simulink model "statdynamic"  (R2019b)
settings: Solver=ode45  StartTime=0.0  StopTime=100  MaxStep=0.0001  RelTol=1e-3
libraries: simulink x5
settings Model: Creator=Roman  LastModifiedBy=romak

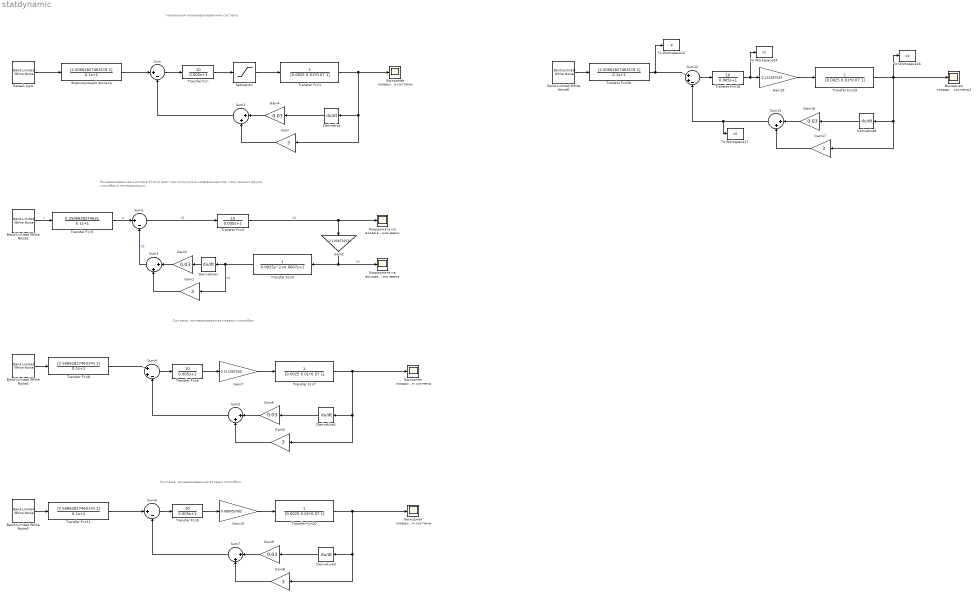
== system statdynamic ==
  note: Система, линеаризованная первым способом
  note: Начальная нелинеаризованная система
  note: Линеаризованная система
      | K(лин) взят как полусумма коэффециентов, полученных двумя способами линеаризации
  note: Система, линеаризованная вторым способом
  Band-Limited White Noise{1..3,6} (4 alike) : simulink/Sources/Band-Limited White Noise  Cov=[1]  Ts=0.0001  seed=[23341]
  Derivative{,1..3,6} (5 alike) : Derivative  CoefficientInTFapproximation=1
  Gain{,1,5,8,17} (5 alike) : Gain  Gain=3
  Gain10 : Gain  Gain=0.089352492
  Gain{3..4,6,9,18} (5 alike) : Gain  Gain=0.03
  Gain19 : Gain  Gain=0.112397533
  Gain2 : Gain  Gain=0.100875013
  Gain7 : Gain  Gain=0.112397533
  Saturation : Saturate  UpperLimit=pi/6  LowerLimit=-pi/6
  Sum : Sum  Inputs=|+-
  Sum1 : Sum  Inputs=|+-
  Sum12 : Sum  Inputs=|++-
  Sum{2..3,5,7,13} (5 alike) : Sum  Inputs=|++
  Sum4 : Sum  Inputs=|++-
  Sum6 : Sum  Inputs=|+-
  To Workspace12 : ToWorkspace  VariableName=e  SampleTime=-1
  To Workspace14 : ToWorkspace  VariableName=x2  SampleTime=-1
  To Workspace16 : ToWorkspace  VariableName=x4  SampleTime=-1
  To Workspace17 : ToWorkspace  VariableName=x5  SampleTime=-1
  Transfer Fcn{,3,6,9,18} (5 alike) : TransferFcn  Numerator=[10]  Denominator=[0.005 1]
  Transfer Fcn{1,7,10,19} (4 alike) : TransferFcn  Denominator=[0.0025 0.01*0.07 1]
  Transfer Fcn11 : TransferFcn  Numerator=[2.506628274631*0.1]  Denominator=[0.1 1]
  Transfer Fcn20 : TransferFcn  Numerator=[2.506628274631*0.1]  Denominator=[0.1 1]
  Transfer Fcn4 : TransferFcn  Denominator=[0.0025 0.0007 1]
  Transfer Fcn5 : TransferFcn  Numerator=[0.2506628274631]  Denominator=[0.1 1]
  Transfer Fcn8 : TransferFcn  Numerator=[2.506628274631*0.1]  Denominator=[0.1 1]
  "Белый шум " : simulink/Sources/Band-Limited White Noise  Cov=[1]  Ts=0.0001  seed=[23341]
  Выходная координата линеаризованной вторым способом системы : Scope
  Выходная координата линеаризованной первым способом системы : Scope
  Выходная координата линеаризованной первым способом системы2 : Scope
  Выходная координата системы : Scope
  "Координата на входе в линеаризованное звено " : Scope
  Координата на выходе из линеаризованного звена : Scope
  "Формирующий фильтр " : TransferFcn  Numerator=[2.506628274631*0.1]  Denominator=[0.1 1]
  wires:
  Derivative/1 -> Gain4/1
  Sum/1 -> Transfer Fcn/1
  Saturation/1 -> Transfer Fcn1/1
  Transfer Fcn1/1 -> Выходная координата системы/1, Gain/1, Derivative/1
  Transfer Fcn/1 -> Saturation/1
  Gain/1 -> Sum2/2
  Sum2/1 -> Sum/2
  "Белый шум "/1 -> "Формирующий фильтр "/1
  "Формирующий фильтр "/1 -> Sum/1
  Gain1/1 -> Sum3/2
  Band-Limited White Noise1/1 -> Transfer Fcn5/1  "v"
  Transfer Fcn3/1 -> "Координата на входе в линеаризованное звено "/1, Gain2/1  "X2"
  Sum1/1 -> Transfer Fcn3/1  "X1"
  Transfer Fcn5/1 -> Sum1/1  "xi"
  Gain2/1 -> Координата на выходе из линеаризованного звена/1, Transfer Fcn4/1  "X3"
  Transfer Fcn4/1 -> Gain1/1, Derivative1/1  "X4"
  Derivative1/1 -> Gain3/1
  Sum3/1 -> Sum1/2  "X5"
  Gain3/1 -> Sum3/1
  Gain4/1 -> Sum2/1
  Gain5/1 -> Sum5/2
  Band-Limited White Noise2/1 -> Transfer Fcn8/1
  Transfer Fcn6/1 -> Gain7/1
  Sum4/1 -> Transfer Fcn6/1
  Transfer Fcn8/1 -> Sum4/1
  Gain7/1 -> Transfer Fcn7/1
  Derivative2/1 -> Gain6/1
  Sum5/1 -> Sum4/3
  Transfer Fcn7/1 -> Выходная координата линеаризованной первым способом системы/1, Gain5/1, Derivative2/1
  Gain6/1 -> Sum5/1
  Transfer Fcn9/1 -> Gain10/1
  Gain10/1 -> Transfer Fcn10/1
  Band-Limited White Noise3/1 -> Transfer Fcn11/1
  Transfer Fcn10/1 -> Выходная координата линеаризованной вторым способом системы/1, Gain8/1, Derivative3/1
  Gain9/1 -> Sum7/1
  Derivative3/1 -> Gain9/1
  Transfer Fcn11/1 -> Sum6/1
  Gain8/1 -> Sum7/2
  Sum6/1 -> Transfer Fcn9/1
  Sum7/1 -> Sum6/2
  Transfer Fcn19/1 -> Выходная координата линеаризованной первым способом системы2/1, Gain17/1, Derivative6/1, To Workspace16/1
  Sum13/1 -> To Workspace17/1, Sum12/3
  Gain19/1 -> Transfer Fcn19/1
  Gain18/1 -> Sum13/1
  Gain17/1 -> Sum13/2
  Sum12/1 -> Transfer Fcn18/1
  Band-Limited White Noise6/1 -> Transfer Fcn20/1
  Transfer Fcn20/1 -> To Workspace12/1, Sum12/1
  Transfer Fcn18/1 -> To Workspace14/1, Gain19/1
  Derivative6/1 -> Gain18/1
